simulink model "GetStartModel"  (R2026a)
settings: Solver=VariableStepAuto  StopTime=10000/200e6
undefined symbols (not defined in the file): cospi
settings Model: Creator=jiemingx  LastModifiedBy=jiemingx
settings DebuggingCC: MergeDetectMultiDrivingBlocksExec=error
settings ModelReferenceCC: PropagateSignalLabelsOutOfModel=on

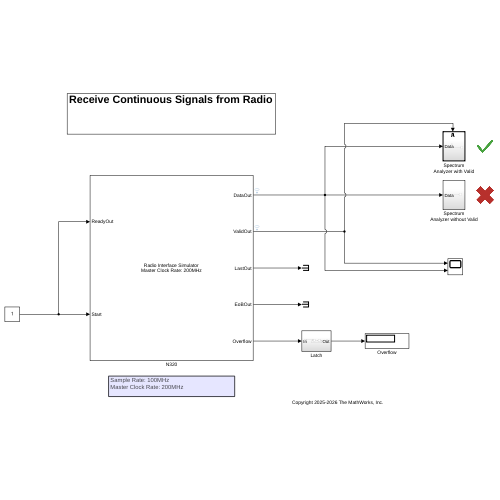
[thumbnail: Simulink's stored preview of the top-level diagram]
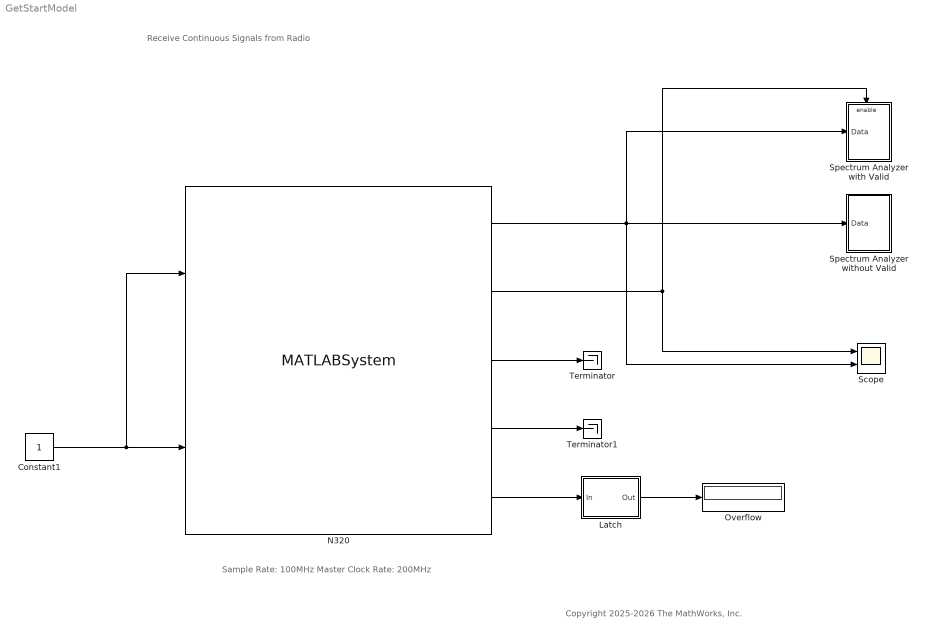
== system GetStartModel ==
  note: Receive Continuous Signals from Radio
  note: Sample Rate: 100MHz
      | Master Clock Rate: 200MHz
  note: Copyright 2025-2026 The MathWorks, Inc.
  Constant1 : Constant  OutDataTypeStr=boolean  SampleTime=1/200e6
  Latch : Subsystem
  N320 : MATLABSystem  System=RadioInterfaceSim  Device=N320  TXRX=RX  ClockSource=Radio  SampleRate=100e6  DUTClockRate=120e6  InputDataSource=cospi((0:10000)/5)  SimulateUsing=Interpreted execution  ClockUncertainty=off  Uncertainty=0  Jitter=0
      mask Type: RadioInterfaceSim
  Overflow : Display
  Scope : Scope  NumInputPorts=2
      settings: ActiveDisplayYMinimum=-0.21703295494266084  ActiveDisplayYMaximum=1.5720024082707651
  Spectrum Analyzer with Valid : Subsystem
  Spectrum Analyzer without Valid : Subsystem
  Terminator : Terminator
  Terminator1 : Terminator
  wires:
  Latch/1(Out) -> Overflow/1
  N320/1 -> Spectrum Analyzer without Valid/1(Data), Spectrum Analyzer with Valid/1(Data), Scope/2
  N320/2 -> Spectrum Analyzer with Valid/Enable, Scope/1
  Constant1/1 -> N320/1, N320/2
  N320/3 -> Terminator/1
  N320/4 -> Terminator1/1
  N320/5 -> Latch/1(In)

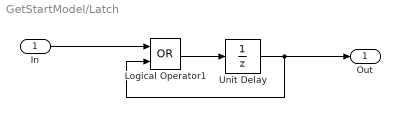
== system GetStartModel/Latch ==
  In : Inport
  Logical Operator1 : Logic  Operator=OR  AllPortsSameDT=off  OutDataTypeStr=boolean
  Unit Delay : UnitDelay  SampleTime=-1
  Out : Outport
  wires:
  Unit Delay/1 -> Out/1, Logical Operator1/2
  In/1 -> Logical Operator1/1
  Logical Operator1/1 -> Unit Delay/1

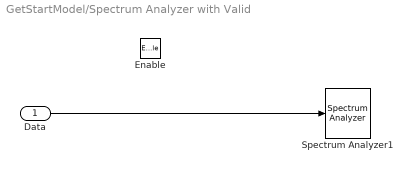
== system GetStartModel/Spectrum Analyzer with Valid ==
  Data : Inport
  Enable : EnablePort
  Spectrum Analyzer1 : SpectrumAnalyzer  WindowPosition=[1518.000000,680.000000,800.000000,500.000000,]  ScopeFrameLocation=window  SampleRateSource=Property  SampleRate=100e6  WindowInvariantSamplesPerUpdate=on  YLimits=[-41.4493 28.5653]
  wires:
  Data/1 -> Spectrum Analyzer1/1

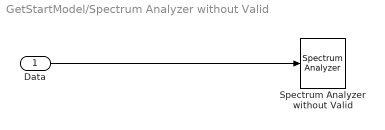
== system GetStartModel/Spectrum Analyzer without Valid ==
  Data : Inport
  Spectrum Analyzer without Valid : SpectrumAnalyzer  WindowPosition=[1491.000000,141.000000,800.000000,500.000000,]  ScopeFrameLocation=window  SampleRateSource=Property  SampleRate=100e6  WindowInvariantSamplesPerUpdate=on  YLimits=[-45.7486 30.7136]  ExpandToolstrip=on  SelectedToolstripTab=spectrumAnalyzerToolstrip.measurementsTab
  wires:
  Data/1 -> Spectrum Analyzer without Valid/1
